simulink model "MCU_CmdTransV2"  (R2022b)
settings: Solver=FixedStepDiscrete  StartTime=0.0  StopTime=10.0  FixedStep=0.001  RelTol=1e-3
undefined symbols (not defined in the file or in its folder): ANALOG, cCurrentLoopMode, cNoneMode, cTorqueLoopMode, ParamCfg_CommandSource_u16, TESTBED, VEHICLE
libraries: simulink x4
settings Model: DataDictionary=MCU_CmdTransV2_objects.sldd  Creator=ZYH  LastModifiedBy=ZYH
settings OptimizationCC: DefaultParameterBehavior=Inlined  EnhancedBackFolding=on  PassReuseOutputArgsAs=Individual arguments  OptimizeBlockOrder=speed  DifferentSizesBufferReuse=on  OptimizationCustomize=off  EfficientTunableParamExpr=on
settings DebuggingCC: ParameterTunabilityLossMsg=error
settings SFSimCC: MATLABDynamicMemAlloc=off
settings RTWCC: Description=Embedded Coder  SystemTargetFile=ert.tlc  GenCodeOnly=on  TemplateMakefile=ert_default_tmf
settings CodeAppCC: ForceParamTrailComments=on  IgnoreCustomStorageClasses=off  OperatorAnnotations=on  SimulinkDataObjDesc=on  SFDataObjDesc=on  InsertBlockDesc=on
settings ERTTargetCC: TargetLangStandard=C99 (ISO)  GenerateSampleERTMain=on  InlinedParameterPlacement=NonHierarchical  ERTCustomFileTemplate=example_file_process.tlc

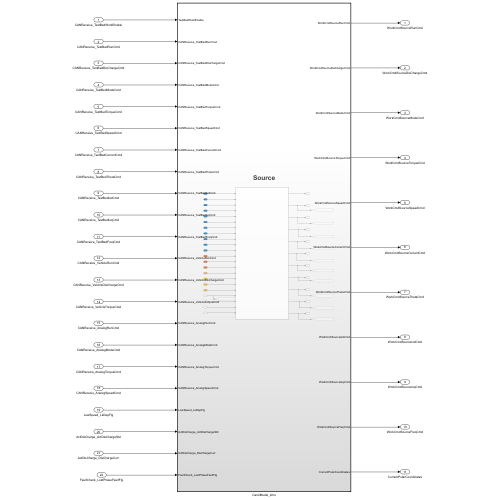
[thumbnail: Simulink's stored preview of the top-level diagram]
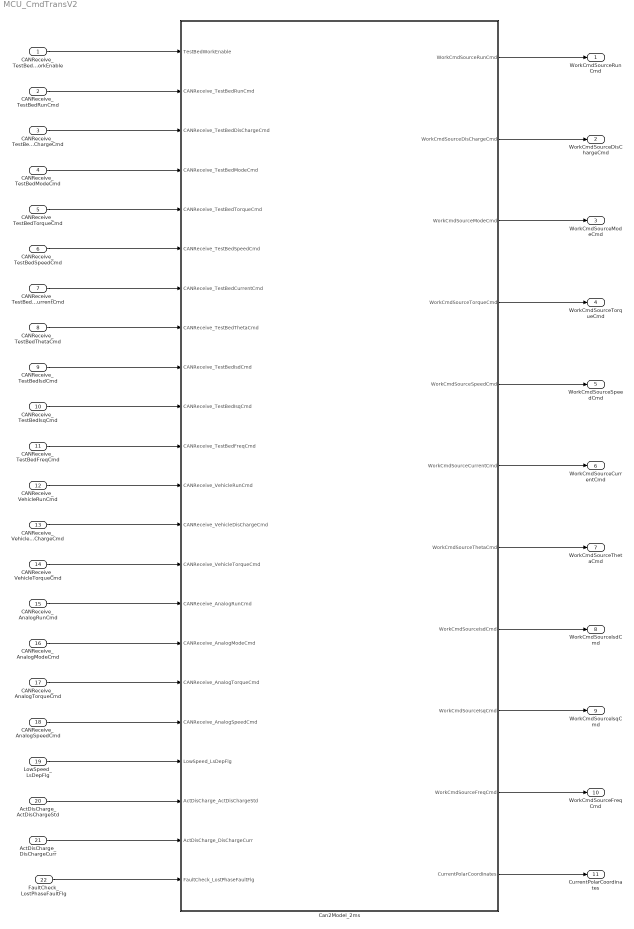
== system MCU_CmdTransV2 ==
  CANReceive_TestBedWorkEnable : Inport
  CANReceive_TestBedRunCmd : Inport  Port=2
  CANReceive_TestBedDisChargeCmd : Inport  Port=3
  CANReceive_TestBedModeCmd : Inport  Port=4
  CANReceive_TestBedTorqueCmd : Inport  Port=5
  CANReceive_TestBedSpeedCmd : Inport  Port=6
  CANReceive_TestBedCurrentCmd : Inport  Port=7
  CANReceive_TestBedThetaCmd : Inport  Port=8
  CANReceive_TestBedIsdCmd : Inport  Port=9
  CANReceive_TestBedIsqCmd : Inport  Port=10
  CANReceive_TestBedFreqCmd : Inport  Port=11
  CANReceive_VehicleRunCmd : Inport  Port=12
  CANReceive_VehicleDisChargeCmd : Inport  Port=13
  CANReceive_VehicleTorqueCmd : Inport  Port=14
  CANReceive_AnalogRunCmd : Inport  Port=15
  CANReceive_AnalogModeCmd : Inport  Port=16
  CANReceive_AnalogTorqueCmd : Inport  Port=17
  CANReceive_AnalogSpeedCmd : Inport  Port=18
  LowSpeed_LsDepFlg : Inport  Port=19
  ActDisCharge_ActDisChargeStd : Inport  Port=20
  ActDisCharge_DisChargeCurr : Inport  Port=21
  FaultCheck_LostPhaseFaultFlg : Inport  Port=22
  Can2Model_2ms : Subsystem  TreatAsAtomicUnit=on
  WorkCmdSourceRunCmd : Outport
  WorkCmdSourceDisChargeCmd : Outport  Port=2
  WorkCmdSourceModeCmd : Outport  Port=3
  WorkCmdSourceTorqueCmd : Outport  Port=4
  WorkCmdSourceSpeedCmd : Outport  Port=5
  WorkCmdSourceCurrentCmd : Outport  Port=6
  WorkCmdSourceThetaCmd : Outport  Port=7
  WorkCmdSourceIsdCmd : Outport  Port=8
  WorkCmdSourceIsqCmd : Outport  Port=9
  WorkCmdSourceFreqCmd : Outport  Port=10
  CurrentPolarCoordinates : Outport  Port=11
  wires:
  CANReceive_TestBedModeCmd/1 -> Can2Model_2ms/4(CANReceive_TestBedModeCmd)
  CANReceive_TestBedTorqueCmd/1 -> Can2Model_2ms/5(CANReceive_TestBedTorqueCmd)
  CANReceive_TestBedDisChargeCmd/1 -> Can2Model_2ms/3(CANReceive_TestBedDisChargeCmd)
  CANReceive_TestBedWorkEnable/1 -> Can2Model_2ms/1(TestBedWorkEnable)
  CANReceive_TestBedRunCmd/1 -> Can2Model_2ms/2(CANReceive_TestBedRunCmd)
  CANReceive_TestBedIsdCmd/1 -> Can2Model_2ms/9(CANReceive_TestBedIsdCmd)
  CANReceive_TestBedIsqCmd/1 -> Can2Model_2ms/10(CANReceive_TestBedIsqCmd)
  CANReceive_TestBedThetaCmd/1 -> Can2Model_2ms/8(CANReceive_TestBedThetaCmd)
  CANReceive_TestBedFreqCmd/1 -> Can2Model_2ms/11(CANReceive_TestBedFreqCmd)
  CANReceive_VehicleRunCmd/1 -> Can2Model_2ms/12(CANReceive_VehicleRunCmd)
  CANReceive_VehicleDisChargeCmd/1 -> Can2Model_2ms/13(CANReceive_VehicleDisChargeCmd)
  CANReceive_TestBedCurrentCmd/1 -> Can2Model_2ms/7(CANReceive_TestBedCurrentCmd)
  CANReceive_TestBedSpeedCmd/1 -> Can2Model_2ms/6(CANReceive_TestBedSpeedCmd)
  CANReceive_AnalogTorqueCmd/1 -> Can2Model_2ms/17(CANReceive_AnalogTorqueCmd)
  CANReceive_AnalogSpeedCmd/1 -> Can2Model_2ms/18(CANReceive_AnalogSpeedCmd)
  CANReceive_AnalogModeCmd/1 -> Can2Model_2ms/16(CANReceive_AnalogModeCmd)
  LowSpeed_LsDepFlg/1 -> Can2Model_2ms/19(LowSpeed_LsDepFlg)
  CANReceive_AnalogRunCmd/1 -> Can2Model_2ms/15(CANReceive_AnalogRunCmd)
  CANReceive_VehicleTorqueCmd/1 -> Can2Model_2ms/14(CANReceive_VehicleTorqueCmd)
  ActDisCharge_ActDisChargeStd/1 -> Can2Model_2ms/20(ActDisCharge_ActDisChargeStd)
  ActDisCharge_DisChargeCurr/1 -> Can2Model_2ms/21(ActDisCharge_DisChargeCurr)
  FaultCheck_LostPhaseFaultFlg/1 -> Can2Model_2ms/22(FaultCheck_LostPhaseFaultFlg)
  Can2Model_2ms/1(WorkCmdSourceRunCmd) -> WorkCmdSourceRunCmd/1
  Can2Model_2ms/2(WorkCmdSourceDisChargeCmd) -> WorkCmdSourceDisChargeCmd/1
  Can2Model_2ms/3(WorkCmdSourceModeCmd) -> WorkCmdSourceModeCmd/1
  Can2Model_2ms/4(WorkCmdSourceTorqueCmd) -> WorkCmdSourceTorqueCmd/1
  Can2Model_2ms/5(WorkCmdSourceSpeedCmd) -> WorkCmdSourceSpeedCmd/1
  Can2Model_2ms/6(WorkCmdSourceCurrentCmd) -> WorkCmdSourceCurrentCmd/1
  Can2Model_2ms/7(WorkCmdSourceThetaCmd) -> WorkCmdSourceThetaCmd/1
  Can2Model_2ms/8(WorkCmdSourceIsdCmd) -> WorkCmdSourceIsdCmd/1
  Can2Model_2ms/9(WorkCmdSourceIsqCmd) -> WorkCmdSourceIsqCmd/1
  Can2Model_2ms/11(CurrentPolarCoordinates) -> CurrentPolarCoordinates/1
  Can2Model_2ms/10(WorkCmdSourceFreqCmd) -> WorkCmdSourceFreqCmd/1

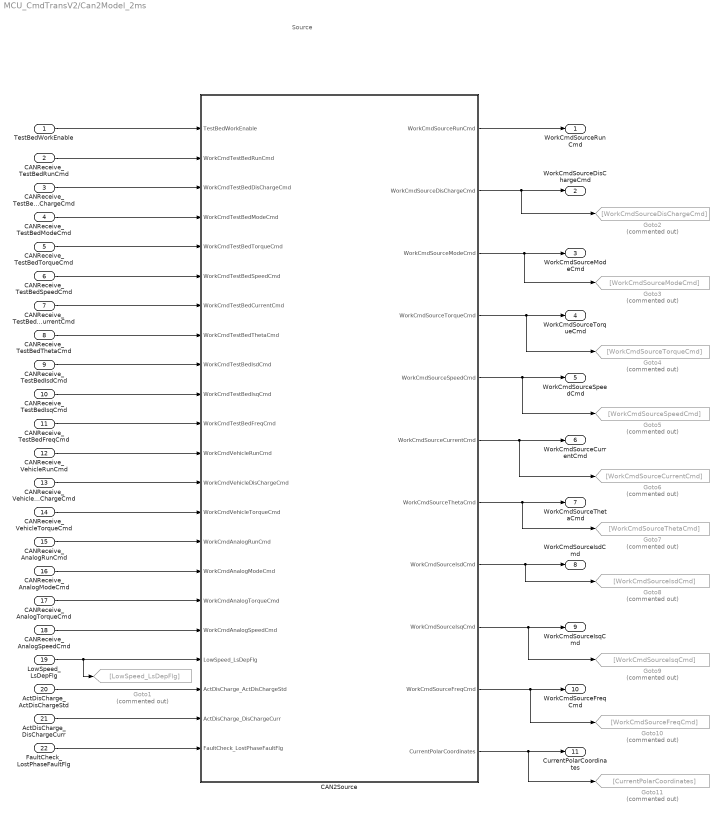
== system MCU_CmdTransV2/Can2Model_2ms ==
  note: Source
  TestBedWorkEnable : Inport
  CANReceive_TestBedRunCmd : Inport  Port=2
  CANReceive_TestBedDisChargeCmd : Inport  Port=3
  CANReceive_TestBedModeCmd : Inport  Port=4
  CANReceive_TestBedTorqueCmd : Inport  Port=5
  CANReceive_TestBedSpeedCmd : Inport  Port=6
  CANReceive_TestBedCurrentCmd : Inport  Port=7
  CANReceive_TestBedThetaCmd : Inport  Port=8
  CANReceive_TestBedIsdCmd : Inport  Port=9
  CANReceive_TestBedIsqCmd : Inport  Port=10
  CANReceive_TestBedFreqCmd : Inport  Port=11
  CANReceive_VehicleRunCmd : Inport  Port=12
  CANReceive_VehicleDisChargeCmd : Inport  Port=13
  CANReceive_VehicleTorqueCmd : Inport  Port=14
  CANReceive_AnalogRunCmd : Inport  Port=15
  CANReceive_AnalogModeCmd : Inport  Port=16
  CANReceive_AnalogTorqueCmd : Inport  Port=17
  CANReceive_AnalogSpeedCmd : Inport  Port=18
  LowSpeed_LsDepFlg : Inport  Port=19
  ActDisCharge_ActDisChargeStd : Inport  Port=20
  ActDisCharge_DisChargeCurr : Inport  Port=21
  FaultCheck_LostPhaseFaultFlg : Inport  Port=22
  CAN2Source : Subsystem  TreatAsAtomicUnit=on
      settings: RTWSystemCode=Nonreusable function
  Goto1 : Goto  Commented=on  GotoTag=LowSpeed_LsDepFlg
  Goto10 : Goto  Commented=on  GotoTag=WorkCmdSourceFreqCmd
  Goto11 : Goto  Commented=on  GotoTag=CurrentPolarCoordinates
  Goto2 : Goto  Commented=on  GotoTag=WorkCmdSourceDisChargeCmd
  Goto3 : Goto  Commented=on  GotoTag=WorkCmdSourceModeCmd
  Goto4 : Goto  Commented=on  GotoTag=WorkCmdSourceTorqueCmd
  Goto5 : Goto  Commented=on  GotoTag=WorkCmdSourceSpeedCmd
  Goto6 : Goto  Commented=on  GotoTag=WorkCmdSourceCurrentCmd
  Goto7 : Goto  Commented=on  GotoTag=WorkCmdSourceThetaCmd
  Goto8 : Goto  Commented=on  GotoTag=WorkCmdSourceIsdCmd
  Goto9 : Goto  Commented=on  GotoTag=WorkCmdSourceIsqCmd
  WorkCmdSourceRunCmd : Outport
  WorkCmdSourceDisChargeCmd : Outport  Port=2
  WorkCmdSourceModeCmd : Outport  Port=3
  WorkCmdSourceTorqueCmd : Outport  Port=4
  WorkCmdSourceSpeedCmd : Outport  Port=5
  WorkCmdSourceCurrentCmd : Outport  Port=6
  WorkCmdSourceThetaCmd : Outport  Port=7
  WorkCmdSourceIsdCmd : Outport  Port=8
  WorkCmdSourceIsqCmd : Outport  Port=9
  WorkCmdSourceFreqCmd : Outport  Port=10
  CurrentPolarCoordinates : Outport  Port=11
  wires:
  CANReceive_TestBedTorqueCmd/1 -> CAN2Source/5(WorkCmdTestBedTorqueCmd)
  CANReceive_TestBedIsdCmd/1 -> CAN2Source/9(WorkCmdTestBedIsdCmd)
  CANReceive_TestBedIsqCmd/1 -> CAN2Source/10(WorkCmdTestBedIsqCmd)
  LowSpeed_LsDepFlg/1 -> Goto1/1, CAN2Source/19(LowSpeed_LsDepFlg)
  FaultCheck_LostPhaseFaultFlg/1 -> CAN2Source/22(FaultCheck_LostPhaseFaultFlg)
  CANReceive_AnalogModeCmd/1 -> CAN2Source/16(WorkCmdAnalogModeCmd)
  CANReceive_AnalogTorqueCmd/1 -> CAN2Source/17(WorkCmdAnalogTorqueCmd)
  CAN2Source/5(WorkCmdSourceSpeedCmd) -> Goto5/1, WorkCmdSourceSpeedCmd/1
  CANReceive_VehicleTorqueCmd/1 -> CAN2Source/14(WorkCmdVehicleTorqueCmd)
  CANReceive_VehicleRunCmd/1 -> CAN2Source/12(WorkCmdVehicleRunCmd)
  ActDisCharge_DisChargeCurr/1 -> CAN2Source/21(ActDisCharge_DisChargeCurr)
  CANReceive_TestBedCurrentCmd/1 -> CAN2Source/7(WorkCmdTestBedCurrentCmd)
  CANReceive_TestBedFreqCmd/1 -> CAN2Source/11(WorkCmdTestBedFreqCmd)
  CAN2Source/10(WorkCmdSourceFreqCmd) -> WorkCmdSourceFreqCmd/1, Goto10/1
  CAN2Source/3(WorkCmdSourceModeCmd) -> Goto3/1, WorkCmdSourceModeCmd/1
  CAN2Source/7(WorkCmdSourceThetaCmd) -> Goto7/1, WorkCmdSourceThetaCmd/1
  CANReceive_AnalogSpeedCmd/1 -> CAN2Source/18(WorkCmdAnalogSpeedCmd)
  CANReceive_TestBedRunCmd/1 -> CAN2Source/2(WorkCmdTestBedRunCmd)
  CAN2Source/4(WorkCmdSourceTorqueCmd) -> Goto4/1, WorkCmdSourceTorqueCmd/1
  CANReceive_VehicleDisChargeCmd/1 -> CAN2Source/13(WorkCmdVehicleDisChargeCmd)
  TestBedWorkEnable/1 -> CAN2Source/1(TestBedWorkEnable)
  CANReceive_TestBedDisChargeCmd/1 -> CAN2Source/3(WorkCmdTestBedDisChargeCmd)
  CAN2Source/11(CurrentPolarCoordinates) -> Goto11/1, CurrentPolarCoordinates/1
  CANReceive_AnalogRunCmd/1 -> CAN2Source/15(WorkCmdAnalogRunCmd)
  CANReceive_TestBedThetaCmd/1 -> CAN2Source/8(WorkCmdTestBedThetaCmd)
  CAN2Source/9(WorkCmdSourceIsqCmd) -> Goto9/1, WorkCmdSourceIsqCmd/1
  ActDisCharge_ActDisChargeStd/1 -> CAN2Source/20(ActDisCharge_ActDisChargeStd)
  CAN2Source/1(WorkCmdSourceRunCmd) -> WorkCmdSourceRunCmd/1
  CAN2Source/6(WorkCmdSourceCurrentCmd) -> Goto6/1, WorkCmdSourceCurrentCmd/1
  CANReceive_TestBedModeCmd/1 -> CAN2Source/4(WorkCmdTestBedModeCmd)
  CAN2Source/2(WorkCmdSourceDisChargeCmd) -> Goto2/1, WorkCmdSourceDisChargeCmd/1
  CAN2Source/8(WorkCmdSourceIsdCmd) -> Goto8/1, WorkCmdSourceIsdCmd/1
  CANReceive_TestBedSpeedCmd/1 -> CAN2Source/6(WorkCmdTestBedSpeedCmd)

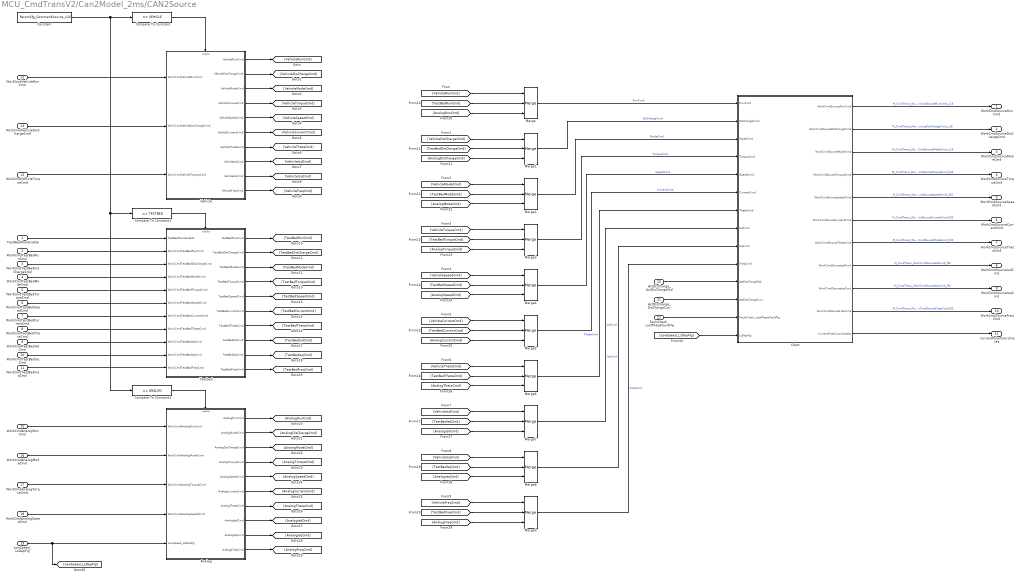
== system MCU_CmdTransV2/Can2Model_2ms/CAN2Source ==
  TestBedWorkEnable : Inport
  WorkCmdTestBedRunCmd : Inport  Port=2
  WorkCmdTestBedDisChargeCmd : Inport  Port=3
  WorkCmdTestBedModeCmd : Inport  Port=4
  WorkCmdTestBedTorqueCmd : Inport  Port=5
  WorkCmdTestBedSpeedCmd : Inport  Port=6
  WorkCmdTestBedCurrentCmd : Inport  Port=7
  WorkCmdTestBedThetaCmd : Inport  Port=8
  WorkCmdTestBedIsdCmd : Inport  Port=9
  WorkCmdTestBedIsqCmd : Inport  Port=10
  WorkCmdTestBedFreqCmd : Inport  Port=11
  WorkCmdVehicleRunCmd : Inport  Port=12
  WorkCmdVehicleDisChargeCmd : Inport  Port=13
  WorkCmdVehicleTorqueCmd : Inport  Port=14
  WorkCmdAnalogRunCmd : Inport  Port=15
  WorkCmdAnalogModeCmd : Inport  Port=16
  WorkCmdAnalogTorqueCmd : Inport  Port=17
  WorkCmdAnalogSpeedCmd : Inport  Port=18
  LowSpeed_LsDepFlg : Inport  Port=19
  ActDisCharge_ActDisChargeStd : Inport  Port=20
  ActDisCharge_DisChargeCurr : Inport  Port=21
  FaultCheck_LostPhaseFaultFlg : Inport  Port=22
  Analog : Subsystem  TreatAsAtomicUnit=on
  Chart : Stateflow chart  TreatAsAtomicUnit=on
  Compare To Constant : simulink/Logic and Bit Operations/Compare To Constant  relop===  const=VEHICLE  OutDataTypeStr=boolean
  Compare To Constant1 : simulink/Logic and Bit Operations/Compare To Constant  relop===  const=TESTBED  OutDataTypeStr=boolean
  Compare To Constant2 : simulink/Logic and Bit Operations/Compare To Constant  relop===  const=ANALOG  OutDataTypeStr=boolean
  Constant : Constant  Value=ParamCfg_CommandSource_u16
  Merge{,1..9} (10 alike) : Merge  Inputs=3
  Testbed : Subsystem  TreatAsAtomicUnit=on
  Vehicle : Subsystem
  WorkCmdSourceRunCmd : Outport
  WorkCmdSourceDisChargeCmd : Outport  Port=2
  WorkCmdSourceModeCmd : Outport  Port=3
  WorkCmdSourceTorqueCmd : Outport  Port=4
  WorkCmdSourceSpeedCmd : Outport  Port=5
  WorkCmdSourceCurrentCmd : Outport  Port=6
  WorkCmdSourceThetaCmd : Outport  Port=7
  WorkCmdSourceIsdCmd : Outport  Port=8
  WorkCmdSourceIsqCmd : Outport  Port=9
  WorkCmdSourceFreqCmd : Outport  Port=10
  CurrentPolarCoordinates : Outport  Port=11
  wires:
  Constant/1 -> Compare To Constant2/1, Compare To Constant1/1, Compare To Constant/1
  Compare To Constant/1 -> Vehicle/Enable
  WorkCmdVehicleRunCmd/1 -> Vehicle/1(WorkCmdVehicleRunCmd)
  WorkCmdVehicleDisChargeCmd/1 -> Vehicle/2(WorkCmdVehicleDisChargeCmd)
  WorkCmdVehicleTorqueCmd/1 -> Vehicle/3(WorkCmdVehicleTorqueCmd)
  Compare To Constant1/1 -> Testbed/Enable
  WorkCmdTestBedModeCmd/1 -> Testbed/4(WorkCmdTestBedModeCmd)
  WorkCmdTestBedTorqueCmd/1 -> Testbed/5(WorkCmdTestBedTorqueCmd)
  WorkCmdTestBedDisChargeCmd/1 -> Testbed/3(WorkCmdTestBedDisChargeCmd)
  WorkCmdTestBedSpeedCmd/1 -> Testbed/6(WorkCmdTestBedSpeedCmd)
  WorkCmdTestBedRunCmd/1 -> Testbed/2(WorkCmdTestBedRunCmd)
  WorkCmdTestBedCurrentCmd/1 -> Testbed/7(WorkCmdTestBedCurrentCmd)
  WorkCmdTestBedThetaCmd/1 -> Testbed/8(WorkCmdTestBedThetaCmd)
  WorkCmdTestBedIsdCmd/1 -> Testbed/9(WorkCmdTestBedIsdCmd)
  WorkCmdTestBedIsqCmd/1 -> Testbed/10(WorkCmdTestBedIsqCmd)
  WorkCmdTestBedFreqCmd/1 -> Testbed/11(WorkCmdTestBedFreqCmd)
  Compare To Constant2/1 -> Analog/Enable
  WorkCmdAnalogRunCmd/1 -> Analog/1(WorkCmdAnalogRunCmd)
  WorkCmdAnalogModeCmd/1 -> Analog/2(WorkCmdAnalogModeCmd)
  WorkCmdAnalogTorqueCmd/1 -> Analog/3(WorkCmdAnalogTorqueCmd)
  WorkCmdAnalogSpeedCmd/1 -> Analog/4(WorkCmdAnalogSpeedCmd)
  TestBedWorkEnable/1 -> Testbed/1(TestBedWorkEnable)
  Vehicle/1(VehicleRunCmd) -> [VehicleRunCmd]
  Vehicle/2(VehicleDisChargeCmd) -> [VehicleDisChargeCmd]
  Vehicle/3(VehicleModeCmd) -> [VehicleModeCmd]
  Vehicle/4(VehicleTorqueCmd) -> [VehicleTorqueCmd]
  Vehicle/5(VehicleSpeedCmd) -> [VehicleSpeedCmd]
  Vehicle/6(VehicleCurrentCmd) -> [VehicleCurrentCmd]
  Vehicle/7(VehicleThetaCmd) -> [VehicleThetaCmd]
  Vehicle/8(VehicleIsdCmd) -> [VehicleIsdCmd]
  Vehicle/9(VehicleIsqCmd) -> [VehicleIsqCmd]
  Vehicle/10(VehicleFreqCmd) -> [VehicleFreqCmd]
  Testbed/2(TestBedDisChargeCmd) -> [TestBedDisChargeCmd]
  Testbed/3(TestBedModeCmd) -> [TestBedModeCmd]
  Testbed/4(TestBedTorqueCmd) -> [TestBedTorqueCmd]
  Testbed/5(TestBedSpeedCmd) -> [TestBedSpeedCmd]
  Testbed/6(TestBedCurrentCmd) -> [TestBedCurrentCmd]
  Testbed/7(TestBedThetaCmd) -> [TestBedThetaCmd]
  Testbed/8(TestBedIsdCmd) -> [TestBedIsdCmd]
  Testbed/9(TestBedIsqCmd) -> [TestBedIsqCmd]
  Testbed/10(TestBedFreqCmd) -> [TestBedFreqCmd]
  Testbed/1(TestBedRunCmd) -> [TestBedRunCmd]
  Analog/2(AnalogModeCmd) -> [AnalogDisChargeCmd]
  Analog/3(AnalogDisChargeCmd) -> [AnalogModeCmd]
  Analog/4(AnalogTorqueCmd) -> [AnalogTorqueCmd]
  Analog/5(AnalogSpeedCmd) -> [AnalogSpeedCmd]
  Analog/6(AnalogCurrentCmd) -> [AnalogCurrentCmd]
  Analog/7(AnalogThetaCmd) -> [AnalogThetaCmd]
  Analog/8(AnalogIsdCmd) -> [AnalogIsdCmd]
  Analog/9(AnalogIsqCmd) -> [AnalogIsqCmd]
  Analog/10(AnalogFreqCmd) -> [AnalogFreqCmd]
  Analog/1(AnalogRunCmd) -> [AnalogRunCmd]
  [VehicleRunCmd] -> Merge/1
  [VehicleDisChargeCmd] -> Merge1/1
  [VehicleModeCmd] -> Merge2/1
  [VehicleTorqueCmd] -> Merge3/1
  [VehicleSpeedCmd] -> Merge4/1
  [VehicleFreqCmd] -> Merge9/1
  [VehicleCurrentCmd] -> Merge5/1
  [VehicleThetaCmd] -> Merge6/1
  [VehicleIsdCmd] -> Merge7/1
  [VehicleIsqCmd] -> Merge8/1
  [TestBedRunCmd] -> Merge/2
  [TestBedDisChargeCmd] -> Merge1/2
  [TestBedModeCmd] -> Merge2/2
  [TestBedTorqueCmd] -> Merge3/2
  [TestBedSpeedCmd] -> Merge4/2
  [TestBedCurrentCmd] -> Merge5/2
  [TestBedThetaCmd] -> Merge6/2
  [TestBedIsdCmd] -> Merge7/2
  [TestBedIsqCmd] -> Merge8/2
  [TestBedFreqCmd] -> Merge9/2
  [AnalogFreqCmd] -> Merge9/3
  [AnalogRunCmd] -> Merge/3
  [AnalogDisChargeCmd] -> Merge1/3
  [AnalogModeCmd] -> Merge2/3
  [AnalogTorqueCmd] -> Merge3/3
  [AnalogSpeedCmd] -> Merge4/3
  [AnalogCurrentCmd] -> Merge5/3
  [AnalogThetaCmd] -> Merge6/3
  [AnalogIsdCmd] -> Merge7/3
  [AnalogIsqCmd] -> Merge8/3
  Merge/1 -> Chart/1(RunCmd)  "RunCmd"
  Merge1/1 -> Chart/2(DisChargeCmd)  "DisChargeCmd"
  Merge2/1 -> Chart/3(ModeCmd)  "ModeCmd"
  Merge3/1 -> Chart/4(TorqueCmd)  "TorqueCmd"
  Merge4/1 -> Chart/5(SpeedCmd)  "SpeedCmd"
  Merge5/1 -> Chart/6(CurrentCmd)  "CurrentCmd"
  Merge6/1 -> Chart/7(ThetaCmd)  "ThetaCmd"
  Merge7/1 -> Chart/8(IsdCmd)  "IsdCmd"
  Merge8/1 -> Chart/9(IsqCmd)  "IsqCmd"
  Merge9/1 -> Chart/10(FreqCmd)  "FreqCmd"
  LowSpeed_LsDepFlg/1 -> [LowSpeed_LsDepFlg], Analog/5(LowSpeed_LsDepFlg)
  Chart/1(WorkCmdSourceRunCmd) -> WorkCmdSourceRunCmd/1  "M_CmdTrans_WorkCmdSourceRunCmd_u16"
  Chart/2(WorkCmdSourceDisChargeCmd) -> WorkCmdSourceDisChargeCmd/1  "M_CmdTrans_WorkCmdSourceDisChargeCmd_u16"
  Chart/3(WorkCmdSourceModeCmd) -> WorkCmdSourceModeCmd/1  "M_CmdTrans_WorkCmdSourceModeCmd_u16"
  Chart/4(WorkCmdSourceTorqueCmd) -> WorkCmdSourceTorqueCmd/1  "M_CmdTrans_WorkCmdSourceTorqueCmd_f32"
  Chart/5(WorkCmdSourceSpeedCmd) -> WorkCmdSourceSpeedCmd/1  "M_CmdTrans_WorkCmdSourceSpeedCmd_f32"
  Chart/6(WorkCmdSourceCurrentCmd) -> WorkCmdSourceCurrentCmd/1  "M_CmdTrans_WorkCmdSourceCurrentCmd_f32"
  Chart/7(WorkCmdSourceThetaCmd) -> WorkCmdSourceThetaCmd/1  "M_CmdTrans_WorkCmdSourceThetaCmd_f32"
  Chart/8(WorkCmdSourceIsdCmd) -> WorkCmdSourceIsdCmd/1  "M_CmdTrans_WorkCmdSourceIsdCmd_f32"
  Chart/9(WorkCmdSourceIsqCmd) -> WorkCmdSourceIsqCmd/1  "M_CmdTrans_WorkCmdSourceIsqCmd_f32"
  Chart/10(WorkCmdSourceFreqCmd) -> WorkCmdSourceFreqCmd/1  "M_CmdTrans_WorkCmdSourceFreqCmd_f32"
  ActDisCharge_ActDisChargeStd/1 -> Chart/11(ActDisChargeStd)
  ActDisCharge_DisChargeCurr/1 -> Chart/12(ActDisChargeCurr)
  FaultCheck_LostPhaseFaultFlg/1 -> Chart/13(FaultCheck_LostPhaseFaultFlg)
  [LowSpeed_LsDepFlg] -> Chart/14(LsDepFlg)
  Chart/11(CurrentPolarCoordinates) -> CurrentPolarCoordinates/1

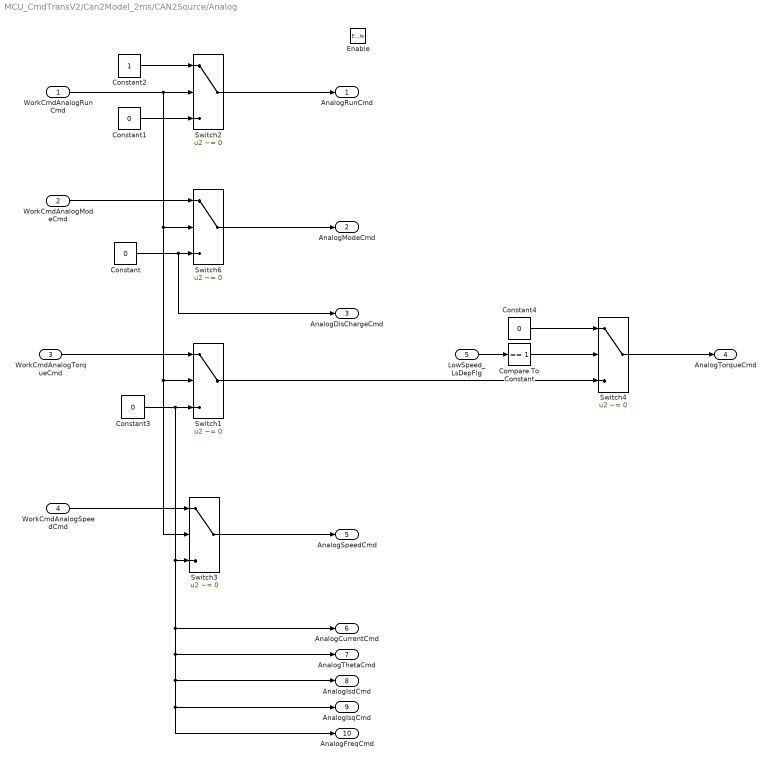
== system MCU_CmdTransV2/Can2Model_2ms/CAN2Source/Analog ==
  WorkCmdAnalogRunCmd : Inport
  WorkCmdAnalogModeCmd : Inport  Port=2
  WorkCmdAnalogTorqueCmd : Inport  Port=3
  WorkCmdAnalogSpeedCmd : Inport  Port=4
  LowSpeed_LsDepFlg : Inport  Port=5
  Enable : EnablePort
  Compare To Constant : simulink/Logic and Bit Operations/Compare To Constant  relop===  const=1  OutDataTypeStr=boolean
  Constant : Constant  Value=0  OutDataTypeStr=uint16
  Constant1 : Constant  Value=0  OutDataTypeStr=uint16
  Constant2 : Constant  OutDataTypeStr=uint16
  Constant3 : Constant  Value=0  OutDataTypeStr=single
  Constant4 : Constant  Value=0  OutDataTypeStr=single
  Switch{1..4,6} (5 alike) : Switch  Criteria=u2 ~= 0  SaturateOnIntegerOverflow=off  InputSameDT=off
  AnalogRunCmd : Outport
  AnalogModeCmd : Outport  Port=2
  AnalogDisChargeCmd : Outport  Port=3
  AnalogTorqueCmd : Outport  Port=4
  AnalogSpeedCmd : Outport  Port=5
  AnalogCurrentCmd : Outport  Port=6
  AnalogThetaCmd : Outport  Port=7
  AnalogIsdCmd : Outport  Port=8
  AnalogIsqCmd : Outport  Port=9
  AnalogFreqCmd : Outport  Port=10
  wires:
  WorkCmdAnalogRunCmd/1 -> Switch2/2, Switch3/2, Switch1/2, Switch6/2
  WorkCmdAnalogModeCmd/1 -> Switch6/1
  Switch6/1 -> AnalogModeCmd/1
  Constant/1 -> AnalogDisChargeCmd/1, Switch6/3
  Switch2/1 -> AnalogRunCmd/1
  Constant1/1 -> Switch2/3
  Constant2/1 -> Switch2/1
  WorkCmdAnalogTorqueCmd/1 -> Switch1/1
  Switch1/1 -> Switch4/3
  WorkCmdAnalogSpeedCmd/1 -> Switch3/1
  Switch3/1 -> AnalogSpeedCmd/1
  Constant3/1 -> AnalogFreqCmd/1, AnalogIsqCmd/1, AnalogIsdCmd/1, AnalogThetaCmd/1, AnalogCurrentCmd/1, Switch3/3, Switch1/3
  LowSpeed_LsDepFlg/1 -> Compare To Constant/1
  Compare To Constant/1 -> Switch4/2
  Switch4/1 -> AnalogTorqueCmd/1
  Constant4/1 -> Switch4/1

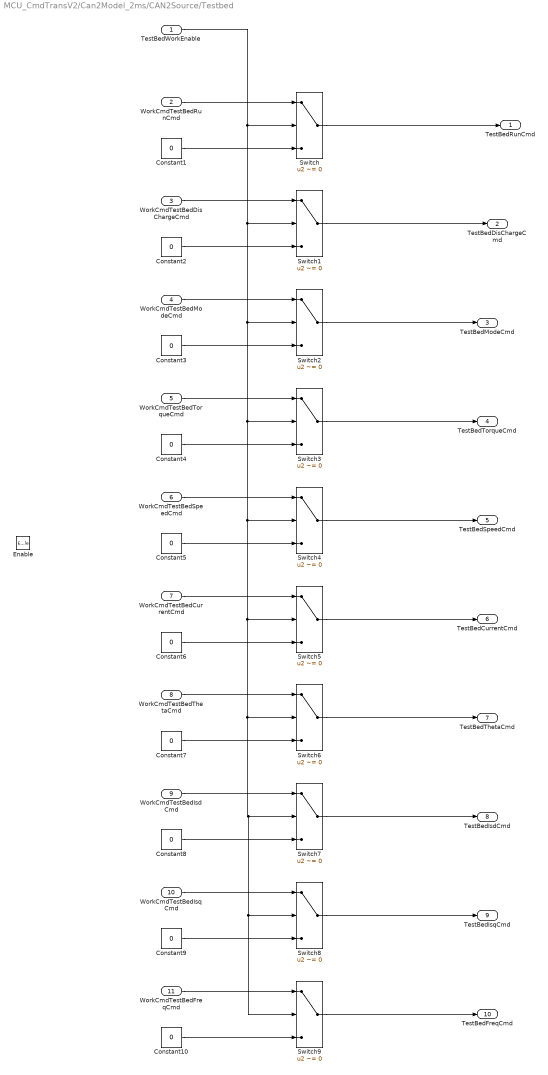
== system MCU_CmdTransV2/Can2Model_2ms/CAN2Source/Testbed ==
  TestBedWorkEnable : Inport
  WorkCmdTestBedRunCmd : Inport  Port=2
  WorkCmdTestBedDisChargeCmd : Inport  Port=3
  WorkCmdTestBedModeCmd : Inport  Port=4
  WorkCmdTestBedTorqueCmd : Inport  Port=5
  WorkCmdTestBedSpeedCmd : Inport  Port=6
  WorkCmdTestBedCurrentCmd : Inport  Port=7
  WorkCmdTestBedThetaCmd : Inport  Port=8
  WorkCmdTestBedIsdCmd : Inport  Port=9
  WorkCmdTestBedIsqCmd : Inport  Port=10
  WorkCmdTestBedFreqCmd : Inport  Port=11
  Enable : EnablePort
  Constant1 : Constant  Value=0  OutDataTypeStr=uint16
  Constant{4..10} (7 alike) : Constant  Value=0  OutDataTypeStr=single
  Constant2 : Constant  Value=0  OutDataTypeStr=uint16
  Constant3 : Constant  Value=0  OutDataTypeStr=uint16
  Switch{,1..9} (10 alike) : Switch  Criteria=u2 ~= 0  SaturateOnIntegerOverflow=off  InputSameDT=off
  TestBedRunCmd : Outport
  TestBedDisChargeCmd : Outport  Port=2
  TestBedModeCmd : Outport  Port=3
  TestBedTorqueCmd : Outport  Port=4
  TestBedSpeedCmd : Outport  Port=5
  TestBedCurrentCmd : Outport  Port=6
  TestBedThetaCmd : Outport  Port=7
  TestBedIsdCmd : Outport  Port=8
  TestBedIsqCmd : Outport  Port=9
  TestBedFreqCmd : Outport  Port=10
  wires:
  Constant1/1 -> Switch/3
  WorkCmdTestBedRunCmd/1 -> Switch/1
  WorkCmdTestBedDisChargeCmd/1 -> Switch1/1
  Constant2/1 -> Switch1/3
  WorkCmdTestBedModeCmd/1 -> Switch2/1
  Constant3/1 -> Switch2/3
  TestBedWorkEnable/1 -> Switch9/2, Switch8/2, Switch7/2, Switch6/2, Switch5/2, Switch4/2, Switch3/2, Switch2/2, Switch1/2, Switch/2
  WorkCmdTestBedTorqueCmd/1 -> Switch3/1
  Constant4/1 -> Switch3/3
  WorkCmdTestBedSpeedCmd/1 -> Switch4/1
  WorkCmdTestBedCurrentCmd/1 -> Switch5/1
  WorkCmdTestBedThetaCmd/1 -> Switch6/1
  WorkCmdTestBedIsdCmd/1 -> Switch7/1
  WorkCmdTestBedIsqCmd/1 -> Switch8/1
  WorkCmdTestBedFreqCmd/1 -> Switch9/1
  Constant5/1 -> Switch4/3
  Constant6/1 -> Switch5/3
  Constant7/1 -> Switch6/3
  Constant8/1 -> Switch7/3
  Constant9/1 -> Switch8/3
  Constant10/1 -> Switch9/3
  Switch/1 -> TestBedRunCmd/1
  Switch1/1 -> TestBedDisChargeCmd/1
  Switch2/1 -> TestBedModeCmd/1
  Switch3/1 -> TestBedTorqueCmd/1
  Switch4/1 -> TestBedSpeedCmd/1
  Switch5/1 -> TestBedCurrentCmd/1
  Switch6/1 -> TestBedThetaCmd/1
  Switch7/1 -> TestBedIsdCmd/1
  Switch8/1 -> TestBedIsqCmd/1
  Switch9/1 -> TestBedFreqCmd/1

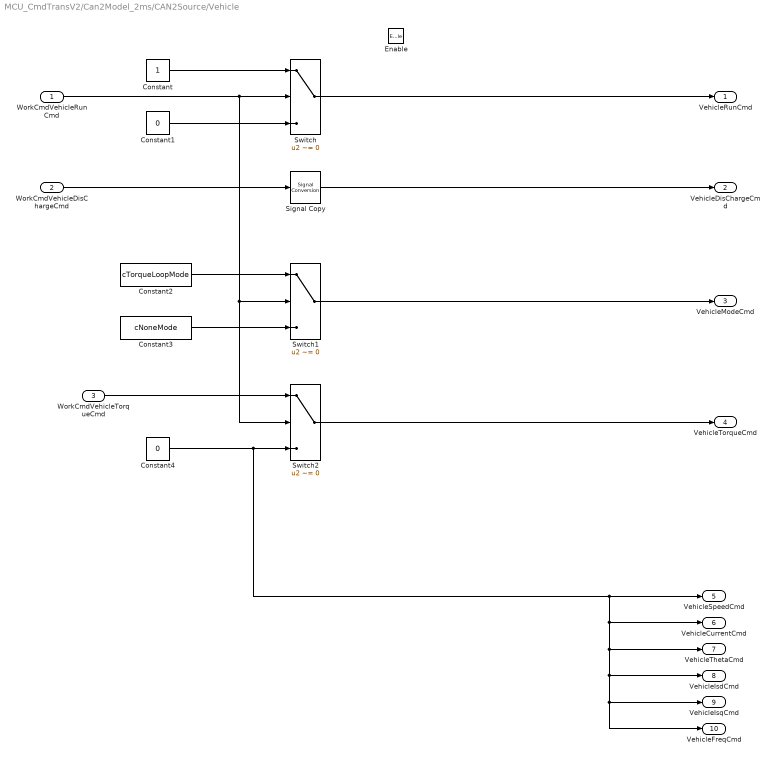
== system MCU_CmdTransV2/Can2Model_2ms/CAN2Source/Vehicle ==
  WorkCmdVehicleRunCmd : Inport
  WorkCmdVehicleDisChargeCmd : Inport  Port=2
  WorkCmdVehicleTorqueCmd : Inport  Port=3
  Enable : EnablePort
  Constant : Constant  OutDataTypeStr=uint16
  Constant1 : Constant  Value=0  OutDataTypeStr=uint16
  Constant2 : Constant  Value=cTorqueLoopMode
  Constant3 : Constant  Value=cNoneMode
  Constant4 : Constant  Value=0  OutDataTypeStr=single
  Signal Copy : SignalConversion  OverrideOpt=off
  Switch : Switch  Criteria=u2 ~= 0  SaturateOnIntegerOverflow=off  InputSameDT=off
  Switch1 : Switch  Criteria=u2 ~= 0  SaturateOnIntegerOverflow=off  InputSameDT=off
  Switch2 : Switch  Criteria=u2 ~= 0  SaturateOnIntegerOverflow=off  InputSameDT=off
  VehicleRunCmd : Outport
  VehicleDisChargeCmd : Outport  Port=2
  VehicleModeCmd : Outport  Port=3
  VehicleTorqueCmd : Outport  Port=4
  VehicleSpeedCmd : Outport  Port=5
  VehicleCurrentCmd : Outport  Port=6
  VehicleThetaCmd : Outport  Port=7
  VehicleIsdCmd : Outport  Port=8
  VehicleIsqCmd : Outport  Port=9
  VehicleFreqCmd : Outport  Port=10
  wires:
  WorkCmdVehicleRunCmd/1 -> Switch2/2, Switch1/2, Switch/2
  Constant/1 -> Switch/1
  Switch/1 -> VehicleRunCmd/1
  Constant1/1 -> Switch/3
  WorkCmdVehicleDisChargeCmd/1 -> Signal Copy/1
  Signal Copy/1 -> VehicleDisChargeCmd/1
  Constant2/1 -> Switch1/1
  Constant3/1 -> Switch1/3
  Switch1/1 -> VehicleModeCmd/1
  WorkCmdVehicleTorqueCmd/1 -> Switch2/1
  Constant4/1 -> VehicleThetaCmd/1, VehicleFreqCmd/1, VehicleIsqCmd/1, VehicleIsdCmd/1, VehicleCurrentCmd/1, VehicleSpeedCmd/1, Switch2/3
  Switch2/1 -> VehicleTorqueCmd/1

== stateflow chart MCU_CmdTransV2/Can2Model_2ms/CAN2Source/Chart ==
  (default) -> (junction 26) : {
      | WorkCmdSourceRunCmd = RunCmd;
      | WorkCmdSourceDisChargeCmd = DisChargeCmd;
      | WorkCmdSourceModeCmd = ModeCmd;
      | WorkCmdSourceTorqueCmd = TorqueCmd;
      | WorkCmdSourceSpeedCmd = SpeedCmd;
      | WorkCmdSourceCurrentCmd = CurrentCmd;
      | WorkCmdSourceThetaCmd = ThetaCmd;
      | WorkCmdSourceIsdCmd = IsdCmd;
      | WorkCmdSourceIsqCmd = IsqCmd;
      | WorkCmdSourceFreqCmd = FreqCmd;
      | }
  (junction 26) -> (junction 28) [order 1] : [LsDepFlg == 1]{WorkCmdSourceTorqueCmd=0}
  (junction 26) -> (junction 28) [order 2]
  (junction 28) -> (junction 31) [order 1] : [FaultCheck_LostPhaseFaultFlg == 1]...
      | {WorkCmdSourceRunCmd = 1;
      | WorkCmdSourceModeCmd = cTorqueLoopMode}
  (junction 28) -> (junction 31) [order 2]
  (junction 31) -> (junction 35) [order 2] : [ActDisChargeStd == 1]...
      | {WorkCmdSourceRunCmd = 1;
      | WorkCmdSourceModeCmd = cCurrentLoopMode;
      | WorkCmdSourceIsdCmd = ActDisChargeCurr;
      | WorkCmdSourceIsqCmd = 0;
      | CurrentPolarCoordinates =0;}
  (junction 31) -> (junction 35) [order 1]
  (junction 35) -> (junction 40)
  data: RunCmd input; WorkCmdSourceRunCmd output uint16 =0; WorkCmdSourceDisChargeCmd output uint16 =0; WorkCmdSourceModeCmd output uint16 =0; WorkCmdSourceTorqueCmd output single =0; WorkCmdSourceSpeedCmd output single =0; WorkCmdSourceCurrentCmd output single =0; WorkCmdSourceThetaCmd output single =0; WorkCmdSourceIsdCmd output single =0; WorkCmdSourceIsqCmd output single =0; WorkCmdSourceFreqCmd output single =0; DisChargeCmd input; ModeCmd input; TorqueCmd input; SpeedCmd input; CurrentCmd input; ThetaCmd input; IsdCmd input; IsqCmd input; FreqCmd input; ActDisChargeStd input; ActDisChargeCurr input; FaultCheck_LostPhaseFaultFlg input; LsDepFlg input; cTorqueLoopMode parameter; cCurrentLoopMode parameter; CurrentPolarCoordinates output uint16 =0
